simulink model "test_RehaMove3_block__MidLevel"  (R2016b)
settings: Solver=FixedStepDiscrete  StartTime=0.0  StopTime=inf  FixedStep=0.1  RelTol=1e-3
libraries: simulink x2, LIB_RehaMove3 x1
settings Model: SimulationMode=external  ExtModeTrigDuration=10000  Creator=constantin  LastModifiedBy=valtin
settings DataIOCC: LimitDataPoints=on  SaveFormat=Array
settings OptimizationCC: ExpressionDepthLimit=2147483647  LifeSpan=1
settings DebuggingCC: UnderspecifiedInitializationDetection=Classic  MergeDetectMultiDrivingBlocksExec=none  SolverPrmCheckMsg=warning  StateNameClashWarn=warning  SFUnexpectedBacktrackingDiag=warning  SFNoUnconditionalDefaultTransitionDiag=warning  SFExecutionAtInitializationDiag=none
settings HardwareCC: ProdBitPerPointer=32  ProdBitPerSizeT=32  ProdBitPerPtrDiffT=32  ProdLargestAtomicFloat=None  ProdIntDivRoundTo=Undefined  ProdEndianess=Unspecified  ProdWordSize=32  ProdHWDeviceType=32-bit Generic
settings ModelReferenceCC: PropagateSignalLabelsOutOfModel=off
settings SFSimCC: SimParseCustomCode=off
settings RTWCC: SystemTargetFile=ert_linux.tlc  MakeCommand=make_rtw OPTS=-DWITH_HW OPTIMIZATION_FLAGS=-O3  TemplateMakefile=ert_linux.tmf  Description=Linux Embedded Coder  TargetLang=C++
settings CodeAppCC: IgnoreCustomStorageClasses=off  CustomSymbolStrType=$N$R$M  InternalIdentifier=Classic
settings STFCustomTargetCC: ModelReferenceCompliant=off  GeneratePreprocessorConditionals=Disable all  CombineOutputUpdateFcns=on  ERTCustomFileBanners=on  SupportComplex=off  RemoveResetFunc=on  SupportVariableSizeSignals=on  MATLABClassNameForMDSCustomization=Simulink.SoftwareTarget.ERTCustomization  GRTInterface=off  SystemTargetFile=ert_linux.tlc
settings ERTTargetCC: ModelReferenceCompliant=off  ParMdlRefBuildCompliant=off  CompOptLevelCompliant=off  ConcurrentExecutionCompliant=off  GeneratePreprocessorConditionals=Disable all  ERTFirstTimeCompliant=off  SupportComplex=off  SupportContinuousTime=on  SupportNonInlinedSFcns=on  SupportVariableSizeSignals=on  ModelStepFunctionPrototypeControlCompliant=off  CPPClassGenCompliant=off  UseToolchainInfoCompliant=off  ExtMode=on  MultiInstanceErrorCode=None  ERTCustomFileTemplate=ert_linux_file_process.tlc  ConvertIfToSwitch=off  SuppressUnreachableDefaultCases=off
settings ConfigComp: CovMetricSettings=dw  CovHtmlReporting=on  CovSaveCumulativeToWorkspaceVar=on  CovSaveSingleToWorkspaceVar=on  CovExternalEMLEnable=off  CovSFcnEnable=off
settings ConfigurationSet: Description=SimMechanics 2G

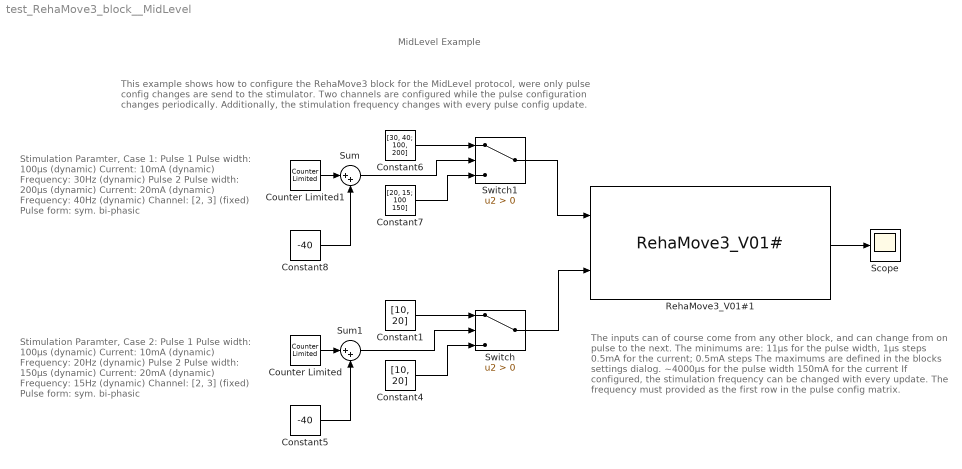
== system test_RehaMove3_block__MidLevel ==
  note: MidLevel Example
  note: This example shows how to configure the RehaMove3 block for the MidLevel protocol, were only pulse config changes are send to the stimulator.
      | Two channels are configured while the pulse configuration changes periodically. Additionally, the stimulation frequency changes with every pulse config update.
  note: Stimulation Paramter, Case 1:
      | Pulse 1
      | Pulse width: 100µs (dynamic)
      | Current: 10mA (dynamic)
      | Frequency: 30Hz (dynamic)
      | Pulse 2
      | Pulse width: 200µs (dynamic)
      | Current: 20mA (dynamic)
      | Frequency: 40Hz (dynamic)
      | Channel: [2, 3] (fixed)
      | Pulse form: sym. bi-phasic
  note: The inputs can of course come from any other block,
      | and can change from on pulse to the next.
      |
      | The minimums are:
      | 11µs for the pulse width, 1µs steps
      | 0.5mA for the current; 0.5mA steps
      |
      | The maximums are defined in the blocks settings dialog.
      | ~4000µs for the pulse width
      | 150mA for the current
      |
      | If configured, the stimulation frequency can be changed with every update.
      | The frequency must provided as the first row in the pulse config matrix.
  note: Stimulation Paramter, Case 2:
      | Pulse 1
      | Pulse width: 100µs (dynamic)
      | Current: 10mA (dynamic)
      | Frequency: 20Hz (dynamic)
      | Pulse 2
      | Pulse width: 150µs (dynamic)
      | Current: 20mA (dynamic)
      | Frequency: 15Hz (dynamic)
      | Channel: [2, 3] (fixed)
      | Pulse form: sym. bi-phasic
  Constant1 : Constant  Value=[10, 20]  OutDataTypeStr=double  SampleTime=-1
  Constant4 : Constant  Value=[10, 20]  OutDataTypeStr=double  SampleTime=-1
  Constant5 : Constant  Value=-40  OutDataTypeStr=double  SampleTime=-1
  Constant6 : Constant  Value=[30, 40; 100, 200]  OutDataTypeStr=double  SampleTime=-1
  Constant7 : Constant  Value=[20, 15; 100 150]  OutDataTypeStr=double  SampleTime=-1
  Constant8 : Constant  Value=-40  OutDataTypeStr=double  SampleTime=-1
  Counter Limited : simulink/Sources/Counter Limited  uplimit=80  tsamp=-1
  Counter Limited1 : simulink/Sources/Counter Limited  uplimit=80  tsamp=-1
  RehaMove3_V01#1 : LIB_RehaMove3/RehaMove3_V01#  stimDevicePath=/dev/ttyUSB0  stimChannels="[ 2  3 ]"  stimFrequency=10  stimRehaMoveProProtocol="Use the MidLevel protocol   -> Only stimulation pulse updates are send."  stimMaxCurrent=90  stimMaxPulsWidth=500  stimBlockID=STIM1  stimTextSampleTime=0.1s (based on stimulation frequency)  SampleTime=0.1  stimThreadInit=on  stimThreadData=on  stimAbortError=3  stimTestAgain=10  llPulseShape=0  llNumberOfParts=1  llMaxStimVoltage=90V  llActivateDenervation=off  mlFStim=20  mlFStimDynamic=on  mlFKeepAlive=1  mlUseSoftStart=on  mlUseRamps=off  mlRampsUpdates=3  mlRampsZeroUpdates=0  miscPrintBlockParam=off  miscPrintDeviceInfos=off  miscPrintSendInfos=off  miscPrintReceiveInfos=off  miscPrintInitInfos=off  miscPrintStimInfos=on  miscPrintRMPInitSettings=on  miscPrintCorrectionChargeWarnings=on  miscPrintSequenceErrors=on  miscPrintTimingErrors=on  miscUseColors=on  miscPrintStats=on  miscEnableAdvancedSettings=off  miscDisableVersionCheck=off
  Scope : Scope
  Sum : Sum  Inputs=|++
  Sum1 : Sum  Inputs=|++
  Switch : Switch  Criteria=u2 > Threshold
  Switch1 : Switch  Criteria=u2 > Threshold
  wires:
  RehaMove3_V01#1/1 -> Scope/1
  Constant1/1 -> Switch/1
  Constant4/1 -> Switch/3
  Sum1/1 -> Switch/2
  Constant6/1 -> Switch1/1
  Constant7/1 -> Switch1/3
  Counter Limited1/1 -> Sum/1
  Sum/1 -> Switch1/2
  Constant8/1 -> Sum/2
  Switch1/1 -> RehaMove3_V01#1/1
  Switch/1 -> RehaMove3_V01#1/2
  Counter Limited/1 -> Sum1/1
  Constant5/1 -> Sum1/2
